simulink model "Pendulum_Sim"  (R2023b)
settings: Solver=VariableStepAuto  StartTime=0.0  StopTime=20.0  RelTol=1e-3
values from neighbouring files (symbols this model uses):
  den1 = [1 0.0307608239168 -157.530949774 -5.39824677832e-15 5.19526995311e-15]    [Phi.mat]    (also in Voltage.mat; Voltage_Filtered.mat; Voltage_Workspace.mat; theta.mat)
  den2 = [1 0.0307608239168 -157.530949774]    [Phi.mat]    (also in Voltage.mat; Voltage_Filtered.mat; Voltage_Workspace.mat; theta.mat)
  den3 = [1 0.0307608239168 -157.530949774 -2.58276315614e-15 2.71416436969e-14]    [Phi.mat]    (also in Voltage.mat; Voltage_Filtered.mat; Voltage_Workspace.mat; theta.mat)
  den4 = [1 0.0307608239168 -157.530949774]    [Phi.mat]    (also in Voltage.mat; Voltage_Filtered.mat; Voltage_Workspace.mat; theta.mat)
  kd = 5    [Model_Adjusted.m]    (also in Model_Simplified.m; Phi.mat; Simulation_model.m = 0.06; Simulation_model_updated.m = 0.15)
  ki = 5    [Model_Adjusted.m]    (also in Model_Simplified.m; Phi.mat; Simulation_model.m = 0; Simulation_model_updated.m = 0)
  kp = 6    [Model_Adjusted.m]    (also in Model_Simplified.m; Phi.mat; Simulation_model.m; Simulation_model_updated.m)
  kt = 0.042    [Model_Adjusted.m]    (also in Model_Simplified.m; Phi.mat; Simulation_model.m; Simulation_model_updated.m)
  Lm = 1.16*10^(-3)    (= 0.00116)    [Model_Adjusted.m]    (also in Model_Simplified.m; Phi.mat; Simulation_model.m = 1.16; Simulation_model_updated.m = 1.16)
  num1 = [0 0 2505.83100187 59.0886717732 -302602.251828]    [Phi.mat]    (also in Voltage.mat; Voltage_Filtered.mat; Voltage_Workspace.mat; theta.mat)
  num2 = [0 0 -2621.93592308]    [Phi.mat]    (also in Voltage.mat; Voltage_Filtered.mat; Voltage_Workspace.mat; theta.mat)
  num3 = [0 0 -2621.93592308 -8.94621646097e-13 -1.71840891779e-13]    [Phi.mat]    (also in Voltage.mat; Voltage_Filtered.mat; Voltage_Workspace.mat; theta.mat)
  num4 = [0 0 11752.8842383]    [Phi.mat]    (also in Voltage.mat; Voltage_Filtered.mat; Voltage_Workspace.mat; theta.mat)
  Rm = 8.4    [Model_Adjusted.m]    (also in Model_Simplified.m; Phi.mat; Simulation_model.m; Simulation_model_updated.m)
libraries: slpidlib x1
settings Model: Creator=Asus  LastModifiedBy=Asus

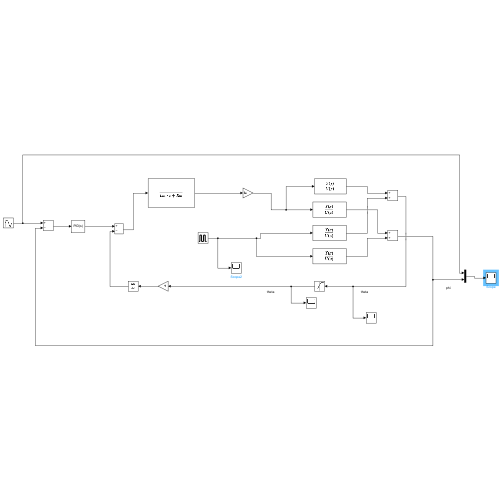
[thumbnail: Simulink's stored preview of the top-level diagram]
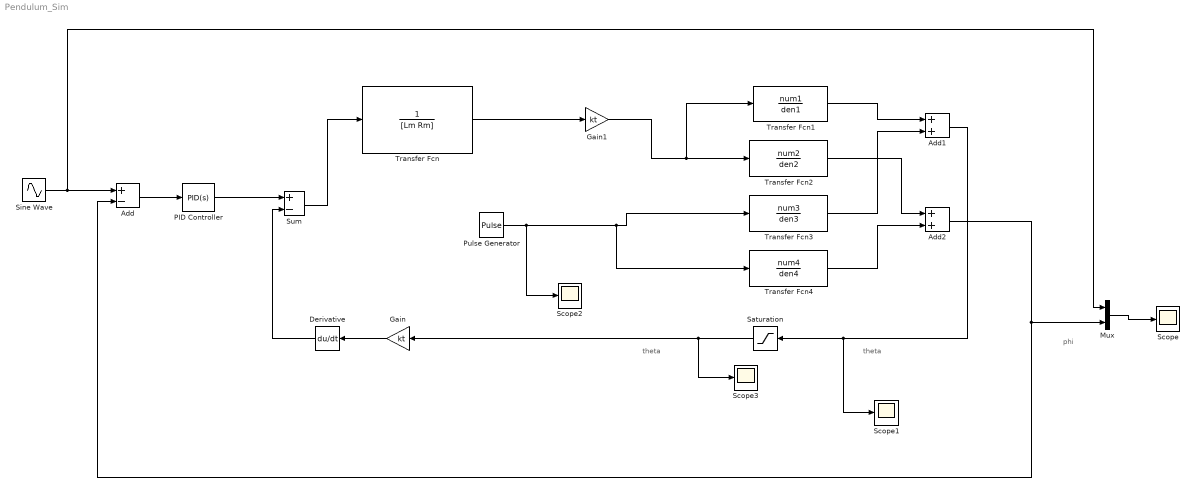
== system Pendulum_Sim ==
  note: phi
  note: theta
  note: theta
  Add : Sum  Inputs=+-
  Add1 : Sum
  Add2 : Sum
  Derivative : Derivative  CoefficientInTFapproximation=0
  Gain : Gain  Gain=kt
  Gain1 : Gain  Gain=kt
  Mux : Mux  Inputs=2
  PID Controller : slpidlib/PID Controller  Controller=PID  Form=Parallel  TimeDomain=Continuous-time  UseExternalTs=off  SampleTime=-1  IntegratorMethod=Forward Euler  FilterMethod=Forward Euler  ControllerParametersSource=internal  P=kp  I=ki  UseKiTs=off  D=kd  N=100  UseFilter=on  TunerSelectOption=Transfer Function Based (PID Tuner App)  InitialConditionSource=internal  InitialConditionForIntegrator=0  InitialConditionForFilter=0  DifferentiatorICPrevScaledInput=0  ExternalReset=none  TrackingMode=off  Kt=1  LimitOutput=off  SatLimitsSource=internal  UpperSaturationLimit=inf  LowerSaturationLimit=-inf  LinearizeAsGain=on  AntiWindupMode=none  Kb=1  LimitIntegrator=off  UpperIntegratorSaturationLimit=inf  LowerIntegratorSaturationLimit=-inf  POutMin=[]  POutMax=[]  IOutMin=[]  IOutMax=[]  DOutMin=[]  DOutMax=[]  NOutMin=[]  NOutMax=[]  SumOutMin=[]  SumOutMax=[]  SaturationOutMin=[]  SaturationOutMax=[]  PParamMin=[]  PParamMax=[]  IParamMin=[]  IParamMax=[]  DParamMin=[]  DParamMax=[]  NParamMin=[]  NParamMax=[]  KbParamMin=[]  KbParamMax=[]  KtParamMin=[]  KtParamMax=[]  KbOutMin=[]  KbOutMax=[]  KtOutMin=[]  KtOutMax=[]  IntegratorOutMin=[]  IntegratorOutMax=[]  FilterOutMin=[]  FilterOutMax=[]  SumI1OutMin=[]  SumI1OutMax=[]  SumI2OutMin=[]  SumI2OutMax=[]  SumI3OutMin=[]  SumI3OutMax=[]  SumI4OutMin=[]  SumI4OutMax=[]  SumDOutMin=[]  SumDOutMax=[]  DifferentiatorOutMin=[]  DifferentiatorOutMax=[]  FilterDiffOutCoefMin=[]  FilterDiffOutCoefMax=[]  ReciprocalOutMin=[]  ReciprocalOutMax=[]  SumDenOutMin=[]  SumDenOutMax=[]  SumNumOutMin=[]  SumNumOutMax=[]  DivideOutMin=[]  DivideOutMax=[]  UdiffTsProdOutMin=[]  UdiffTsProdOutMax=[]  NTsProdOutMin=[]  NTsProdOutMax=[]  UintegralTsProdOutMin=[]  UintegralTsProdOutMax=[]  UngainTsProdOutMin=[]  UngainTsProdOutMax=[]  ClampingZeroOutDataTypeStr=Inherit: Inherit via back propagation  ClampingZeroOutMin=[]  ClampingZeroOutMax=[]  FilterDenConstantOutDataTypeStr=Inherit: Inherit via back propagation  FilterDenConstantOutMin=[]  FilterDenConstantOutMax=[]  PCopyOutDataTypeStr=Inherit: Inherit via back propagation  PCopyOutMin=[]  PCopyOutMax=[]  NCopyOutDataTypeStr=Inherit: Inherit via back propagation  NCopyOutMin=[]  NCopyOutMax=[]  IntegratorContinuousStateAttributes=''  IntegratorStateMustResolveToSignalObject=off  IntegratorRTWStateStorageClass=Auto  FilterContinuousStateAttributes=''  FilterStateMustResolveToSignalObject=off  FilterRTWStateStorageClass=Auto  ParallelPVariant=InternalParameters  IdealPVariant=Disabled  IVariant=InternalParameters  DVariant=InternalParameters  IntegratorVariant=Continuous  SatVariant=Disabled  AWVariant=Passthrough  PCopyVariant=Disabled  TRVariant=Disabled  FdbkBlocksVariant=Forward  IdealPFdbkVariant=Disabled  SatFdbkVariant=Disabled  DerivativeFilterVariant=ContFilter  NVariant=InternalParameters  NCopyVariant=Disabled  FilterICVariant=InternalICsFilter  IntegratorICVariant=InternalICs  ExternalResetVariant=Disabled  TRSumVariant=Passthrough  SumFdbkVariant=Disabled  SumVariant=Sum_PID  TsampFilterVariant=InternalTs  TsampNgainVariant=Passthrough  TsampIntegralVariant=Disabled_SignalSpec  ExternalSaturationOutDataTypeStr=Inherit: Same as second input
  Pulse Generator : DiscretePulseGenerator  PulseType=Time based  Amplitude=0.01  Period=21
  Saturation : Saturate  UpperLimit=pi/2  LowerLimit=-pi/2
  Scope{,1..3} (4 alike) : Scope
  Sine Wave : Sin  Amplitude=0  SampleTime=0
  Sum : Sum  Inputs=+-
  Transfer Fcn : TransferFcn  Denominator=[Lm Rm]
  Transfer Fcn1 : TransferFcn  Numerator=num1  Denominator=den1  ContinuousStateAttributes='theta1'
  Transfer Fcn2 : TransferFcn  Numerator=num2  Denominator=den2
  Transfer Fcn3 : TransferFcn  Numerator=num3  Denominator=den3
  Transfer Fcn4 : TransferFcn  Numerator=num4  Denominator=den4
  wires:
  Sine Wave/1 -> Mux/1, Add/1
  Add/1 -> PID Controller/1
  PID Controller/1 -> Sum/1
  Sum/1 -> Transfer Fcn/1
  Gain/1 -> Derivative/1
  Derivative/1 -> Sum/2
  Gain1/1 -> Transfer Fcn2/1, Transfer Fcn1/1
  Transfer Fcn/1 -> Gain1/1
  Mux/1 -> Scope/1
  Add1/1 -> Saturation/1, Scope1/1
  Transfer Fcn1/1 -> Add1/1
  Transfer Fcn3/1 -> Add1/2
  Transfer Fcn2/1 -> Add2/1
  Transfer Fcn4/1 -> Add2/2
  Pulse Generator/1 -> Scope2/1, Transfer Fcn4/1, Transfer Fcn3/1
  Add2/1 -> Mux/2, Add/2
  Saturation/1 -> Scope3/1, Gain/1
